simulink model "bilateral_control_force_velocity"  (R2018b)
settings: Solver=VariableStepAuto  StartTime=0.0  StopTime=tsim  FixedStep=0.01  RelTol=1e-3
values from neighbouring files (symbols this model uses):
  Bm = 20    [bilateral_control_parameters.m]
  Bs = 20    [bilateral_control_parameters.m]
  Gf = 1    [bilateral_control_parameters.m]
  ke = 100    [bilateral_control_parameters.m]
  kh = 10000    [bilateral_control_parameters.m]
  Mm = 1    [bilateral_control_parameters.m]
  Ms = 1    [bilateral_control_parameters.m]
  td = 0.1    [bilateral_control_parameters.m]
settings Model: Creator=mariorc  LastModifiedBy=mariorc
settings SFSimCC: SimUseLocalCustomCode=off
settings RTWCC: RTWUseLocalCustomCode=off

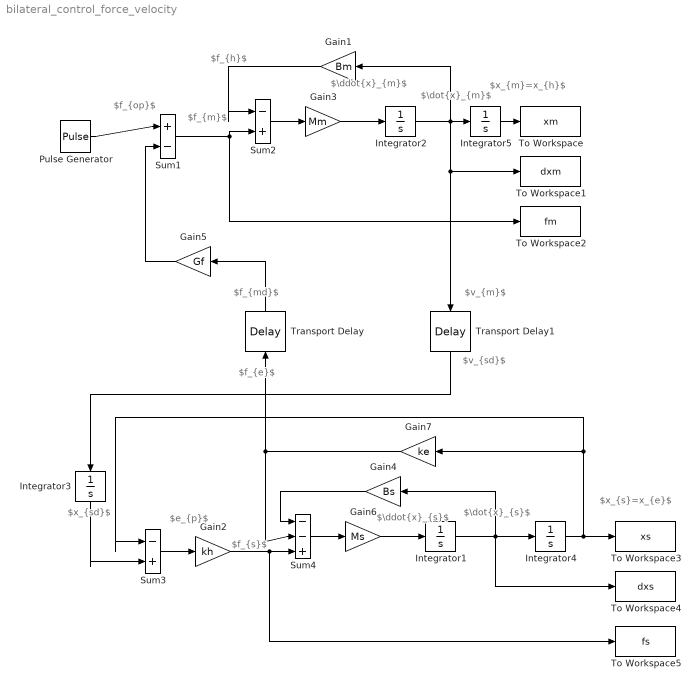
== system bilateral_control_force_velocity ==
  note: $x_{s}=x_{e}$
  note: $f_{s}$
  note: $e_{p}$
  note: $f_{h}$
  note: $x_{m}=x_{h}$
  note: $f_{m}$
  note: $\dot{x}_{m}$
  note: $\dot{x}_{s}$
  note: $f_{md}$
  note: $f_{e}$
  note: $v_{m}$
  note: $v_{sd}$
  note: $f_{op}$
  note: $\ddot{x}_{s}$
  note: $\ddot{x}_{m}$
  note: $x_{sd}$
  Gain1 : Gain  Gain=Bm
  Gain2 : Gain  Gain=kh
  Gain3 : Gain  Gain=Mm
  Gain4 : Gain  Gain=Bs
  Gain5 : Gain  Gain=Gf
  Gain6 : Gain  Gain=Ms
  Gain7 : Gain  Gain=ke
  Integrator{1..5} (5 alike) : Integrator
  Pulse Generator : DiscretePulseGenerator  PulseType=Time based  Period=40  PulseWidth=50
  Sum1 : Sum  Inputs=|+-
  Sum2 : Sum  Inputs=|-+
  Sum3 : Sum  Inputs=|-+
  Sum4 : Sum  Inputs=|--+
  To Workspace : ToWorkspace  VariableName=xm  SaveFormat=Timeseries  SampleTime=-1
  To Workspace1 : ToWorkspace  VariableName=dxm  SaveFormat=Timeseries  SampleTime=-1
  To Workspace2 : ToWorkspace  VariableName=fm  SaveFormat=Timeseries  SampleTime=-1
  To Workspace3 : ToWorkspace  VariableName=xs  SaveFormat=Timeseries  SampleTime=-1
  To Workspace4 : ToWorkspace  VariableName=dxs  SaveFormat=Timeseries  SampleTime=-1
  To Workspace5 : ToWorkspace  VariableName=fs  SaveFormat=Timeseries  SampleTime=-1
  Transport Delay : TransportDelay  DelayTime=td
  Transport Delay1 : TransportDelay  DelayTime=td
  wires:
  Gain5/1 -> Sum1/2
  Gain1/1 -> Sum2/1
  Sum1/1 -> Sum2/2, To Workspace2/1
  Sum2/1 -> Gain3/1
  Gain3/1 -> Integrator2/1
  Integrator2/1 -> Integrator5/1, Gain1/1, To Workspace1/1, Transport Delay1/1
  Pulse Generator/1 -> Sum1/1
  Transport Delay/1 -> Gain5/1
  Gain2/1 -> To Workspace5/1, Sum4/3
  Gain7/1 -> Transport Delay/1, Sum4/2
  Gain6/1 -> Integrator1/1
  Integrator1/1 -> Gain4/1, To Workspace4/1, Integrator4/1
  Integrator4/1 -> Gain7/1, Sum3/1, To Workspace3/1
  Sum4/1 -> Gain6/1
  Gain4/1 -> Sum4/1
  Transport Delay1/1 -> Integrator3/1
  Sum3/1 -> Gain2/1
  Integrator3/1 -> Sum3/2
  Integrator5/1 -> To Workspace/1
